simulink model "piopru_fir_test"  (R2019b)
settings: Solver=FixedStepDiscrete  StartTime=0.0  StopTime=0.01  FixedStep=1e-6  RelTol=1e-3
libraries: aldec_ahdl x2, simulink_extras x1, dspsrcs4 x1
settings Model: Creator=thomas  LastModifiedBy=thomas

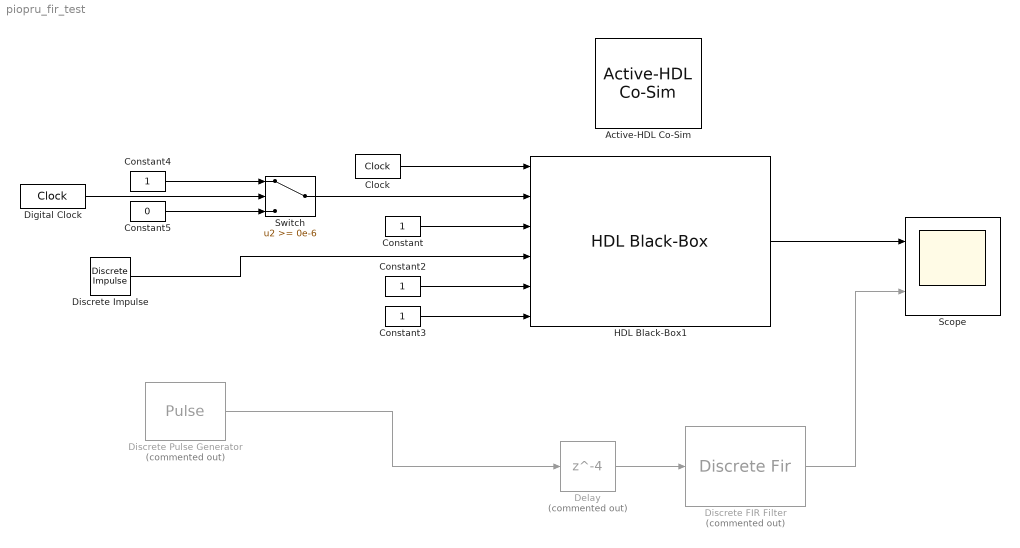
== system piopru_fir_test ==
  Active-HDL Co-Sim : aldec_ahdl/Active-HDL Co-Sim  Tag=Active-HDL_Co-Sim_close  hdl_period=1  hdl_tscale=us  sys_period=[1, 0]  sys_tscale=As In Simulator  cmd_after_vsim=wave -noreg {/piopru_fir_test/\piopru_fir_test/HDL Black-Box1\/data}  wav_fn=$(model_name)  wav_settings=[0,3]  sim_cfg=[1,0,0]  dbg=off  auto_start=on  gen_tb=[0,1,15]  batch_sim=off  tb_fn=$(model_name).log  metavalue_map=[0,0]  sim_resolution=[1,0,1]  active_page=2  aws_en=off  ahdl_en=off  blk_ver=10.5a.RTM  macro_en=[0,0,0]
      settings: SourceProductName=Active-HDL Toolbox
  Clock : simulink_extras/Flip Flops/Clock  period=6e-6
  Constant{,2..4} (4 alike) : Constant
  Constant5 : Constant  Value=0
  Delay : Delay  Commented=on  DelayLength=4  InitialCondition=0  SampleTime=6e-6
  Digital Clock : DigitalClock  SampleTime=1e-6
  Discrete Pulse Generator : DiscretePulseGenerator  Commented=on  Amplitude=127  Period=10  SampleTime=6e-6
  Discrete Impulse : dspsrcs4/Discrete  Impulse  Delay=100  SampleTime=6e-6  FrameSample=1  OutputFrames=off  dataType=double  isSigned=on  wordLen=16  udDataType=sfix(16)  fracBitsMode=Best precision  numFracBits=15  OutDataTypeStr=double  LastOutDataTypeStr=double
  Discrete FIR Filter : DiscreteFir  Commented=on  Coefficients=[127 100 80 127]  SampleTime=6e-6
  HDL Black-Box1 : aldec_ahdl/HDL Black-Box  Tag=Active-HDL_BB_lib  module_m=piopru_fir  ports_cfg={aclk,0,1,2,0,Inherited,8,0,0,0,0,1}{aresetn,0,1,2,0,Inherited,8,0,0,0,0,1}{aclken,0,1,2,0,Inherited,8,0,0,0,0,1}{s_axis_data_tdata,0,-1,2,0,Inherited,0,0,0,0,0,1}{s_axis_data_tvalid,0,1,2,0,Inherited,8,0,0,0,0,1}{m_axis_data_tready,0,1,2,0,Inherited,8,0,0,0,0,1}{s_axis_data_tready,1,1,2,0,1,8,0,0,0,0,1}{m_axis_data_tdata,1,-1,2,0,1,0,0,0,0,0,1}{m_axis_data_tvalid,1,1,2,0,1,8,0,0,0,0,1}  params={AXIS_IQ_TDATA_WIDTH,32,INTEGER}{num_of_coef,51,INTEGER}{coef_size,12,INTEGER}  waves={2,Inputs,2,3,0,15,,-1,-1,-1,0,0,0,0}{0,aclk,0,0,0,15,,-1,-1,-1,0,0,0,0}{0,aresetn,0,0,0,15,,-1,-1,-1,0,0,0,0}{0,aclken,0,0,0,15,,-1,-1,-1,0,0,0,0}{0,s_axis_data_tdata,2,2,0,15,,-1,-1,-1,0,0,0,0}{0,s_axis_data_tvalid,0,0,0,15,,-1,-1,-1,0,0,0,0}{0,m_axis_data_tready,0,0,0,15,,-1,-1,-1,0,0,0,0}{2,Outputs,2,3,0,15,,-1,-1,-1,0,0,0,0}{0,s_axis_data_tready,0,0,0,15,,-1,-1,-1,0,0,0,0}{0,m_axis_data_tdata,2,2,0,100,,-1,-1,-1,1,0,0,0}{0,m_axis_data_tvalid,0,0,0,15,,-1,-1,-1,0,0,0,0}  block_mask=image('HDLBlackBox.jpg','center'); disp('piopru_fir');port_label('input', 1, 'aclk');port_label('input', 2, 'aresetn');port_label('input', 3, 'aclken');port_label('input', 4, 's_axis_data_tdata');port_label('input', 5, 's_axis_data_tvalid');port_label('input', 6, 'm_axis_data_tready');port_label('output', 1, 's_axis_data_tready');port_label('output', 2, 'm_axis_data_tdata');port_label('output', 3, 'm_axis_data_tvalid');  config=[6,3]  inp=[6, 8, 1, 0, 0, 0, 2, 8, 1, 0, 0, 0, 2, 8, 1, 0, 0, 0, 2, 0, abs(32-1 - 0) + 1, 0, 0, 0, 2, 8, 1, 0, 0, 0, 2, 8, 1, 0, 0, 0, 2]  out=[3, 8, 1, 0, 0, 0, 2, 0, abs(32-1 - 0) + 1, 0, 0, 0, 2, 8, 1, 0, 0, 0, 2]  sampling=[1, -1, -1, -1, -1, -1, -1, 1, 1, 1]  active_page={766,476,2,{0,{80,0,0,1},{35,1,2,1},{65,2,2,1},{70,3,2,1},{70,4,2,1},{60,5,2,1},{60,6,2,1},{50,7,2,1},{35,8,2,1},{35,9,2,1},{119,10,0,1}},{1,{106,0,0,1},{55,1,2,1},{70,2,2,1},{75,3,2,1},{75,4,2,1},{45,5,2,1},{45,6,2,1},{45,7,2,1},{165,8,0,1}},{2,{165,0,0,1},{130,1,2,1},{190,2,2,1},{190,3,2,1}},{3,{94,0,0,1},{58,1,2,1},{58,2,2,1},{70,3,2,1},{58,4,2,1}},{4,{83,0,0,1},{70,1,2,1},{80,2,2,1},{50,3,2,1},{50,4,2,1}},{5,{125,0,0,1},{330,1,2,1},{220,2,2,1}},{6,{129,0,0,1},{95,1,1,1},{70,2,2,1},{50,3,1,1},{80,4,1,1},{35,5,2,1},{35,6,2,1},{65,7,0,1},{150,8,0,1}}}  param_val={32,-1,51,-1,12,-1}  clk_val=[0]  ce_val=[0]  blk_ver=10.5a.RTM  blk_conf=0  user_conv=0
      settings: SourceProductName=Active-HDL Toolbox
  Scope : Scope  NumInputPorts=2
  Switch : Switch  Threshold=0e-6
  wires:
  Constant3/1 -> HDL Black-Box1/6
  Discrete FIR Filter/1 -> Scope/2
  Constant2/1 -> HDL Black-Box1/5
  Discrete Pulse Generator/1 -> Delay/1
  Constant4/1 -> Switch/1
  Constant5/1 -> Switch/3
  Digital Clock/1 -> Switch/2
  Switch/1 -> HDL Black-Box1/2
  HDL Black-Box1/2 -> Scope/1
  Delay/1 -> Discrete FIR Filter/1
  Clock/1 -> HDL Black-Box1/1
  Constant/1 -> HDL Black-Box1/3
  Discrete Impulse/1 -> HDL Black-Box1/4
